simulink model "IntegracionExperimental"  (R2023b)
settings: Solver=VariableStepAuto  StartTime=0.0  StopTime=2  RelTol=1e-3
settings Model: Creator=Antonio  LastModifiedBy=Antonio

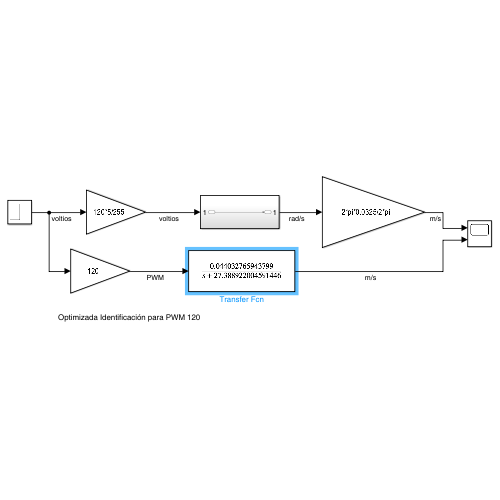
[thumbnail: Simulink's stored preview of the top-level diagram]
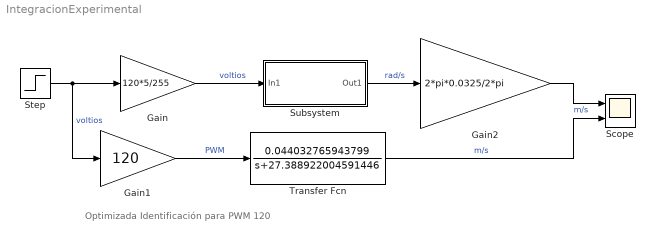
== system IntegracionExperimental ==
  note: Optimizada Identificación para PWM 120
  Gain : Gain  Gain=120*5/255
  Gain1 : Gain  Gain=120
  Gain2 : Gain  Gain=2*pi*0.0325/2*pi
  Scope : Scope  NumInputPorts=2
  Step : Step  SampleTime=0
  Subsystem : Subsystem
  Transfer Fcn : TransferFcn  Numerator=0.044032765943799  Denominator=[1,27.388922004591446]
  wires:
  Step/1 -> Gain1/1, Gain/1  "voltios"
  Subsystem/1(Out1) -> Gain2/1  "rad/s"
  Transfer Fcn/1 -> Scope/2  "m/s"
  Gain1/1 -> Transfer Fcn/1  "PWM"
  Gain/1 -> Subsystem/1(In1)  "voltios"
  Gain2/1 -> Scope/1  "m/s"

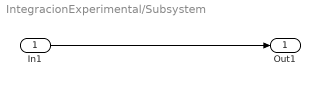
== system IntegracionExperimental/Subsystem ==
  In1 : Inport
  Out1 : Outport
  wires:
  In1/1 -> Out1/1
